simulink model "untitled"  (Simulink 7.4)
settings: Solver=FixedStepDiscrete  StartTime=0.0  StopTime=inf  RelTol=1e-3
undefined symbols (not defined in the file): gray, pause
libraries: vipsnks x2, dspsrcs4 x1, vipsrcs x1, simulink x1, vipanalysis x1
settings Model: Creator=student  LastModifiedBy=student

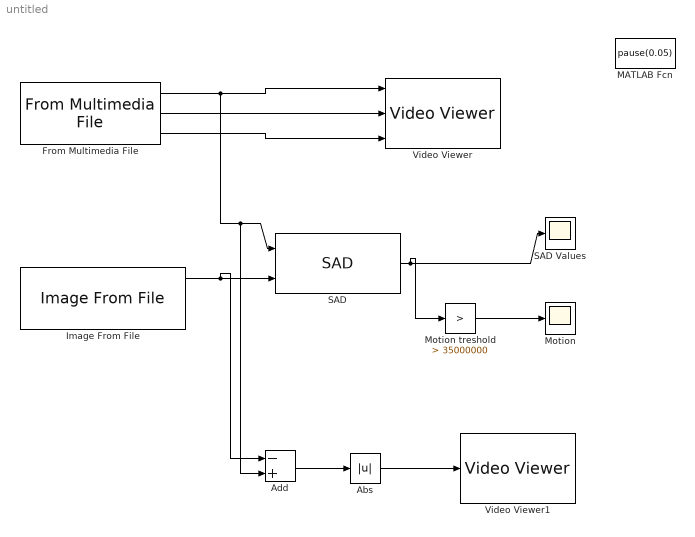
== system untitled ==
  Abs : Abs  OutDataTypeMode=uint8  OutDataType=fixdt(1, 16)  OutScaling=2^0  OutDataTypeStr=uint8
  Add : Sum  Inputs=-+  AccumDataTypeStr=int16  OutDataTypeMode=int16  OutDataType=fixdt(1, 16)  OutScaling=2^-10  OutDataTypeStr=int16
  From Multimedia File : dspsrcs4/From Multimedia File  DialogController=dspDDGCreate  DialogControllerArgs=DataTag0  inputFilename=D:\Multimodal\pn-0930\lab-3\motion1.avi  loop=on  numPlays=inf  outputStreams=Video only  videoDataType=int16  audioDataType=int16  inheritSampleTime=on  userDefinedSampleTime=1/30  noAudioOutput=off  isIntensityVideo=off  colorVideoFormat=Separate color signals  outputEOF=off  dataOrg=Column-major  audioFrameSize=1024
  Image From File : vipsrcs/Image From File  Tag=vipblks_nd  DialogController=vipDDGCreate  DialogControllerArgs=DataTag1  SystemSampleTime=-1  FileName=D:\Multimodal\pn-0930\lab-3\tlo0000.bmp  imagePorts=Separate color signals  Ts=inf  ImageDataType=int16  Signed=on  WordLength=16  sdImageDataType=uint(8)  FractionLengthMode=User-defined  FractionLength=15  OutPortLabels=R|G|B
  MATLAB Fcn : MATLABFcn  MATLABFcn=pause(0.05)  OutputDimensions=0
  Motion : Scope
      settings: YMin=0  YMax=1
  Motion treshold : simulink/Logic and Bit Operations/Compare To Constant  SystemSampleTime=-1  relop=>  const=35000000  LogicOutDataTypeMode=uint8
  SAD : vipanalysis/SAD  DialogController=vipDDGCreate  DialogControllerArgs=DataTag2  output=SAD values  method=Exhaustive  roi=off  invalidROI=Ignore  nearbyPel=off  nearbySize=3  outputMode=Binary point scaling  outputWordLength=32  outputFracLength=0  accumMode=Binary point scaling  accumWordLength=32  accumFracLength=0  roundingMode=Floor  overflowMode=off
  SAD Values : Scope
      settings: YMin=2.5e+007  YMax=8e+007
  Video Viewer : vipsnks/Video Viewer  DialogControllerArgs=DataTag4  inputType=Obsolete7b  imagePorts=Separate color signals  useColorMap=off  colormapValue=gray(256)  specRange=off  minInputVal=0  maxInputVal=255  FigPos=[895 985 410 300]  AxisZoom=on  trueSizedOnce=off  OpenAtMdlStart=on
  Video Viewer1 : vipsnks/Video Viewer  DialogControllerArgs=DataTag6  inputType=Obsolete7b  imagePorts=One multidimensional signal  useColorMap=off  colormapValue=gray(256)  specRange=off  minInputVal=0  maxInputVal=255  FigPos=[867 585 410 300]  AxisZoom=on  trueSizedOnce=off  OpenAtMdlStart=on
  wires:
  From Multimedia File/1 -> Video Viewer/1, SAD/1, Add/2
  From Multimedia File/2 -> Video Viewer/2
  From Multimedia File/3 -> Video Viewer/3
  Image From File/1 -> SAD/2, Add/1
  SAD/1 -> SAD Values/1, Motion treshold/1
  Motion treshold/1 -> Motion/1
  Add/1 -> Abs/1
  Abs/1 -> Video Viewer1/1
